simulink model "AsteroidImpact"  (R2022b)
settings: Solver=ode4  StartTime=0.0  StopTime=45  FixedStep=0.05  RelTol=1e-3
settings Model: Creator=KNMALE002  LastModifiedBy=sohailsingh
settings SolverCC: AlgebraicLoopSolver=TrustRegion
settings DataIOCC: SaveOutput=off  SignalLogging=off  DSMLogging=off  ReturnWorkspaceOutputs=off  TimeSaveName=simulation_time
settings DebuggingCC: UnconnectedInputMsg=warning  UnconnectedOutputMsg=warning  UnconnectedLineMsg=warning  SFMachineParentedDataDiag=warning  ArithmeticOperatorsInVariantConditions=warning
settings ModelReferenceCC: EnableRefExpFcnMdlSchedulingChecks=on
settings SFSimCC: CustomCodeUndefinedFunction=UseInterfaceOnly

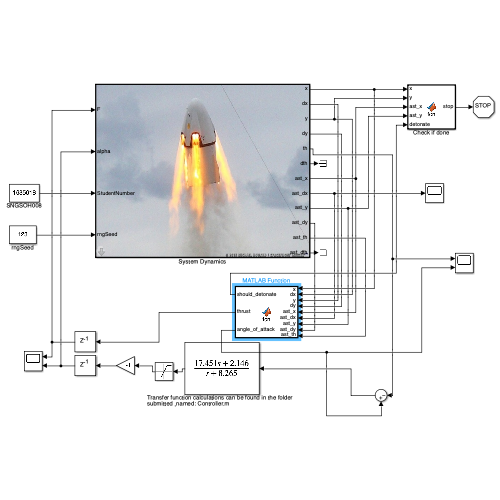
[thumbnail: Simulink's stored preview of the top-level diagram]
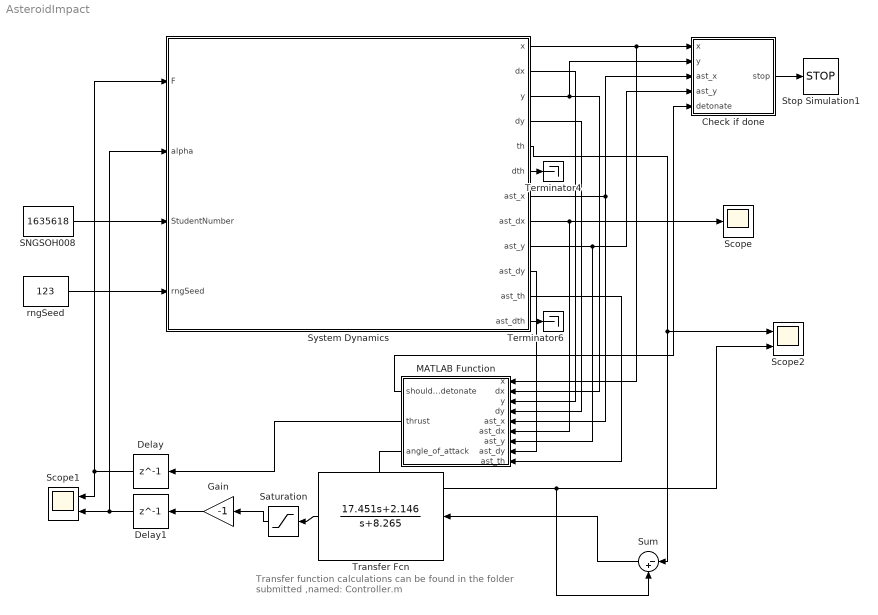
== system AsteroidImpact ==
  note: Transfer function calculations can be found in the folder
      | submitted ,named: Controller.m
  Check if done : MATLAB Function  TreatAsAtomicUnit=on
  Delay : Delay  DelayLength=1  InitialCondition=10000000000
  Delay1 : Delay  DelayLength=1
  Gain : Gain  Gain=-1
  MATLAB Function : MATLAB Function  TreatAsAtomicUnit=on
  SNGSOH008 : Constant  Value=1635618
  Saturation : Saturate  UpperLimit=0.2  LowerLimit=-0.2
  Scope : Scope
  Scope1 : Scope  NumInputPorts=2
  Scope2 : Scope  NumInputPorts=2
  Stop Simulation1 : Stop
  Sum : Sum  Inputs=|-+
  System Dynamics : Subsystem  TreatAsAtomicUnit=on  mask{Value=3}
      mask prompts: Value "Enter mode (1, 2 or 3)"
      mask TypeOptions Value: ScenarioVar/Value
      mask Display: image('lander.jpg');
  Terminator4 : Terminator
  Terminator6 : Terminator
  Transfer Fcn : TransferFcn  Numerator=[17.451 2.146]  Denominator=[1 8.265]
  rngSeed : Constant  Value=123
  wires:
  SNGSOH008/1 -> System Dynamics/3(StudentNumber)
  System Dynamics/1(x) -> MATLAB Function/1(x), Check if done/1(x)
  rngSeed/1 -> System Dynamics/4(rngSeed)
  System Dynamics/3(y) -> MATLAB Function/2(dx), Check if done/2(y)
  System Dynamics/12(ast_dth) -> Terminator6/1
  System Dynamics/7(ast_x) -> MATLAB Function/5(ast_x), Check if done/3(ast_x)
  System Dynamics/9(ast_y) -> Check if done/4(ast_y), MATLAB Function/7(ast_y)
  System Dynamics/8(ast_dx) -> Scope/1, MATLAB Function/6(ast_dx)
  System Dynamics/11(ast_th) -> MATLAB Function/9(ast_th)
  Check if done/1(stop) -> Stop Simulation1/1
  Delay1/1 -> Scope1/2, System Dynamics/2(alpha)
  Delay/1 -> System Dynamics/1(F), Scope1/1
  MATLAB Function/1(should_detonate) -> Check if done/5(detonate)
  System Dynamics/6(dth) -> Terminator4/1
  Saturation/1 -> Gain/1
  Gain/1 -> Delay1/1
  Transfer Fcn/1 -> Saturation/1
  System Dynamics/5(th) -> Sum/1, Scope2/1
  Sum/1 -> Transfer Fcn/1
  MATLAB Function/3(angle_of_attack) -> Sum/2, Scope2/2
  System Dynamics/10(ast_dy) -> MATLAB Function/8(ast_dy)
  MATLAB Function/2(thrust) -> Delay/1
  System Dynamics/2(dx) -> MATLAB Function/3(y)
  System Dynamics/4(dy) -> MATLAB Function/4(dy)

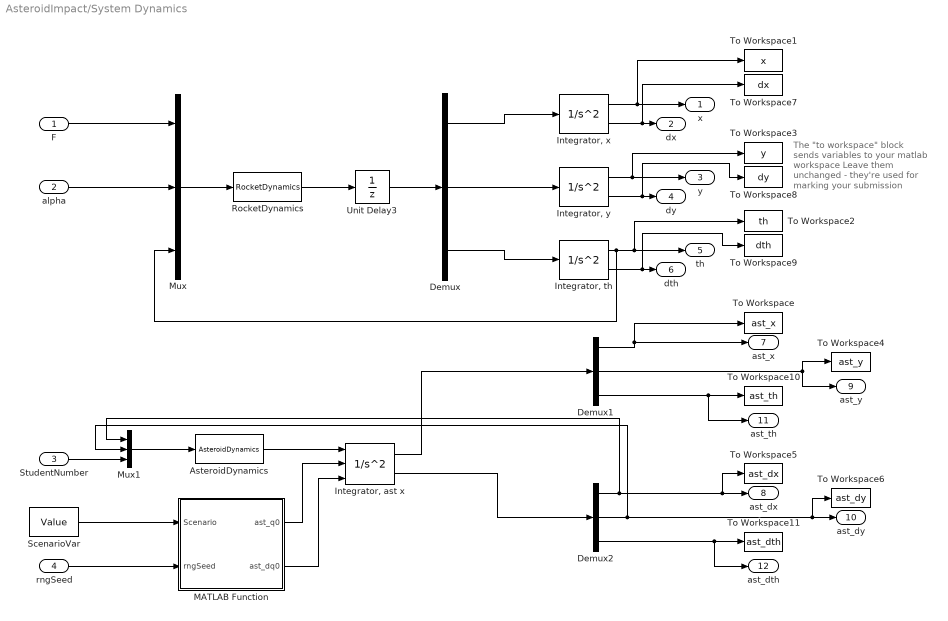
== system AsteroidImpact/System Dynamics ==
  note: The "to workspace" block sends variables to your matlab workspace
      |
      | Leave them unchanged - they're used for marking your submission
  F : Inport
  alpha : Inport  Port=2
  StudentNumber : Inport  Port=3
  rngSeed : Inport  Port=4
  AsteroidDynamics : MATLABFcn  MATLABFcn=AsteroidDynamics  OutputDimensions=3
  Demux : Demux  Outputs=3
  Demux1 : Demux  Outputs=3
  Demux2 : Demux  Outputs=3
  "Integrator, th" : SecondOrderIntegrator  ICX=0  ICDXDT=0
  "Integrator, x" : SecondOrderIntegrator  ICX=0
  "Integrator, y" : SecondOrderIntegrator  ICX=0
  "Integrator, ast x" : SecondOrderIntegrator  ICSourceX=external  ICX=x0  ICSourceDXDT=external
  MATLAB Function : MATLAB Function  TreatAsAtomicUnit=on
  Mux : Mux  Inputs=3
  Mux1 : Mux  Inputs=3
  RocketDynamics : MATLABFcn  MATLABFcn=RocketDynamics  Output1D=off
  ScenarioVar : Constant  Value=Value
  To Workspace : ToWorkspace  VariableName=ast_x  SampleTime=-1
  To Workspace1 : ToWorkspace  VariableName=x  SampleTime=-1
  To Workspace10 : ToWorkspace  VariableName=ast_th  SampleTime=-1
  To Workspace11 : ToWorkspace  VariableName=ast_dth  SampleTime=-1
  To Workspace2 : ToWorkspace  VariableName=th  SampleTime=-1
  To Workspace3 : ToWorkspace  VariableName=y  SampleTime=-1
  To Workspace4 : ToWorkspace  VariableName=ast_y  SampleTime=-1
  To Workspace5 : ToWorkspace  VariableName=ast_dx  SampleTime=-1
  To Workspace6 : ToWorkspace  VariableName=ast_dy  SampleTime=-1
  To Workspace7 : ToWorkspace  VariableName=dx  SampleTime=-1
  To Workspace8 : ToWorkspace  VariableName=dy  SampleTime=-1
  To Workspace9 : ToWorkspace  VariableName=dth  SampleTime=-1
  Unit Delay3 : UnitDelay  SampleTime=-1  HasFrameUpgradeWarning=on
  x : Outport  PortDimensions=1  VectorParamsAs1DForOutWhenUnconnected=off
  dx : Outport  Port=2  PortDimensions=1  VectorParamsAs1DForOutWhenUnconnected=off
  y : Outport  Port=3  PortDimensions=1  VectorParamsAs1DForOutWhenUnconnected=off
  dy : Outport  Port=4  PortDimensions=1  VectorParamsAs1DForOutWhenUnconnected=off
  th : Outport  Port=5  PortDimensions=1  VectorParamsAs1DForOutWhenUnconnected=off
  dth : Outport  Port=6  PortDimensions=1  VectorParamsAs1DForOutWhenUnconnected=off
  ast_x : Outport  Port=7  PortDimensions=1  VectorParamsAs1DForOutWhenUnconnected=off
  ast_dx : Outport  Port=8  PortDimensions=1  VectorParamsAs1DForOutWhenUnconnected=off
  ast_y : Outport  Port=9  PortDimensions=1  VectorParamsAs1DForOutWhenUnconnected=off
  ast_dy : Outport  Port=10  PortDimensions=1  VectorParamsAs1DForOutWhenUnconnected=off
  ast_th : Outport  Port=11  PortDimensions=1  VectorParamsAs1DForOutWhenUnconnected=off
  ast_dth : Outport  Port=12  PortDimensions=1  VectorParamsAs1DForOutWhenUnconnected=off
  wires:
  "Integrator, th"/1 -> th/1, To Workspace2/1, Mux/3
  Demux/1 -> "Integrator, x"/1
  Demux/2 -> "Integrator, y"/1
  Demux/3 -> "Integrator, th"/1
  "Integrator, x"/1 -> x/1, To Workspace1/1
  "Integrator, x"/2 -> To Workspace7/1, dx/1
  "Integrator, y"/2 -> To Workspace8/1, dy/1
  "Integrator, th"/2 -> To Workspace9/1, dth/1
  Mux/1 -> RocketDynamics/1
  RocketDynamics/1 -> Unit Delay3/1
  rngSeed/1 -> MATLAB Function/2(rngSeed)
  ScenarioVar/1 -> MATLAB Function/1(Scenario)
  F/1 -> Mux/1
  alpha/1 -> Mux/2
  Demux1/2 -> To Workspace4/1, ast_y/1
  Demux1/3 -> To Workspace10/1, ast_th/1
  Demux2/3 -> ast_dth/1, To Workspace11/1
  Mux1/1 -> AsteroidDynamics/1
  AsteroidDynamics/1 -> "Integrator, ast x"/1
  "Integrator, ast x"/1 -> Demux1/1
  "Integrator, ast x"/2 -> Demux2/1
  Demux1/1 -> To Workspace/1, ast_x/1
  Demux2/1 -> Mux1/1, To Workspace5/1, ast_dx/1
  Demux2/2 -> Mux1/2, To Workspace6/1, ast_dy/1
  MATLAB Function/1(ast_q0) -> "Integrator, ast x"/2
  MATLAB Function/2(ast_dq0) -> "Integrator, ast x"/3
  StudentNumber/1 -> Mux1/3
  Unit Delay3/1 -> Demux/1
  "Integrator, y"/1 -> y/1, To Workspace3/1

== matlab function AsteroidImpact/System Dynamics/MATLAB Function ==
  data: ast_q0 output; ast_dq0 output; Scenario input; rngSeed input
function [ast_q0, ast_dq0] = fcn(Scenario, rngSeed)
rng(rngSeed);

if (Scenario == 1)
    x0 = -3000;
    y0 =  5000;
    th0 =   0;
    dx0 = 182;
    dy0 = 0;
    dth0 = 0;

elseif (Scenario == 2)
    x0 = -2000 + rand_within_plus_minus(100);
    y0 = 4000 + rand_within_plus_minus(100); 
    th0 = 0;
    dx0 = 170;
    dy0 = 0;
    dth0 = 0.1;

elseif (Scenario == 3)
    x0 = -2500;
    y0 = 3000;
    th0 = 0;
    dx0 = 160;
    dy0 = 100;
    dth0 = deg2rad(rand_within_plus_minus(20)); % rad/sec

else
    error('You entered an invalid mode -- make sure Scenario = 1, 2 or 3')
end

ast_q0  = [ x0;  y0;  th0];
ast_dq0 = [dx0; dy0; dth0];

end

% calling rand_within_plus_minus(100) returns a number between -100 and 100
function n = rand_within_plus_minus(interval)
    n = (rand - 0.5) * 2 * interval;
end

== matlab function AsteroidImpact/MATLAB Function ==
  data: x input; dx input; y input; dy input; ast_x input; ast_dx input; should_detonate output; ast_y input; ast_dy input; thrust output; angle_of_attack output; ast_th input
function [should_detonate, thrust, angle_of_attack] = fcn(x, dx, y, dy, ast_x, ast_dx, ast_y, ast_dy,ast_th)
%Milestone 3 used the framework of milestone 2 with a few alterations. The
%transfer function of the controller was changed to a system on the edge of
%instability which allowed for higher manouverability, alike controllers
%found in fighter jets
% Calculate rocket and asteroid parameters
rocket_pos = [x; y]; % Position of rocket
rocket_vel = [dx; dy]; % Velocity of rocket
thrust = 100000;
asteroid_pos = [ast_x; ast_y]; % Position of asteroid
asteroid_vel = [ast_dx; ast_dy]; % Velocity of asteroid

%The difference in distance between asteroid and rocket is calculated below
% Calculate line of sight 
line_of_sight = asteroid_pos - rocket_pos;

%Desired velocity is calculated using the line of sight calculated above
%and the current position and velocity of the rocket
% Calculate the desired velocity
desired_vel = asteroid_vel + line_of_sight / norm(line_of_sight) * norm(rocket_vel);
desired_heading = atan2(desired_vel(2), desired_vel(1));% the ast_th is chosen as the target point
desired_aoa = desired_heading - ast_th;
 

%The desired velocity and current velocity give the angle of attack
%required
% Calculate angle of attack
angle_of_attack = atan2(desired_vel(2), desired_vel(1)) - atan2(rocket_vel(2), rocket_vel(1));
angle_error = desired_aoa - angle_of_attack;

%PD controller design
Kp = 0.585; % Proportional gain these values are changes and tuned to get a accurate model of the rocket
Kd = 0.001085; % Derivative gain
angle_error = angle_of_attack;
vel_error = desired_vel - rocket_vel;
angle_of_attack = Kp * angle_error + Kd * vel_error(1);
angle_of_attack = max(min(angle_of_attack, pi/2), -pi/2); %AoA is limited to +- 90degs to prevent too sharp turns
%and assists with better control of the rocket

% Collision check - the rocket should detonate based on a single condition
% whether the rocket is within 150m of the rocket
distance_to_asteroid = norm(line_of_sight);
should_detonate = distance_to_asteroid <= 150;

end
%sngsoh008

== matlab function AsteroidImpact/Check if done ==
  data: x input; stop output; y input; ast_x input; ast_y input; detonate input
function stop = fcn(x, y, ast_x, ast_y, detonate)
    % given the signal to detonate
    if detonate == 1
        stop = 1;

    % rocket has hit the asteroid
    elseif norm([x; y] - [ast_x; ast_y]) < 100
        stop = 1;
    
    % rocket has hit the ground OR asteroid is close to they city
    elseif y < 0 || ast_y < 200
        stop = 1;
    
    else
        stop = 0;
    end
end
